simulink model "FinalShape"  (R2020a)
settings: Solver=ode4  StartTime=0.0  StopTime=100  FixedStep=.0001  MaxStep=1e-4  RelTol=1e-3
undefined symbols (not defined in the file or in its folder): kappa_lut_axis, lut_cooling_T, lut_heating_T, sigbuilder_block
settings Model: Creator=nnnmmm  LastModifiedBy=nnnmmm
settings DataIOCC: ExternalInput=sim_input_T

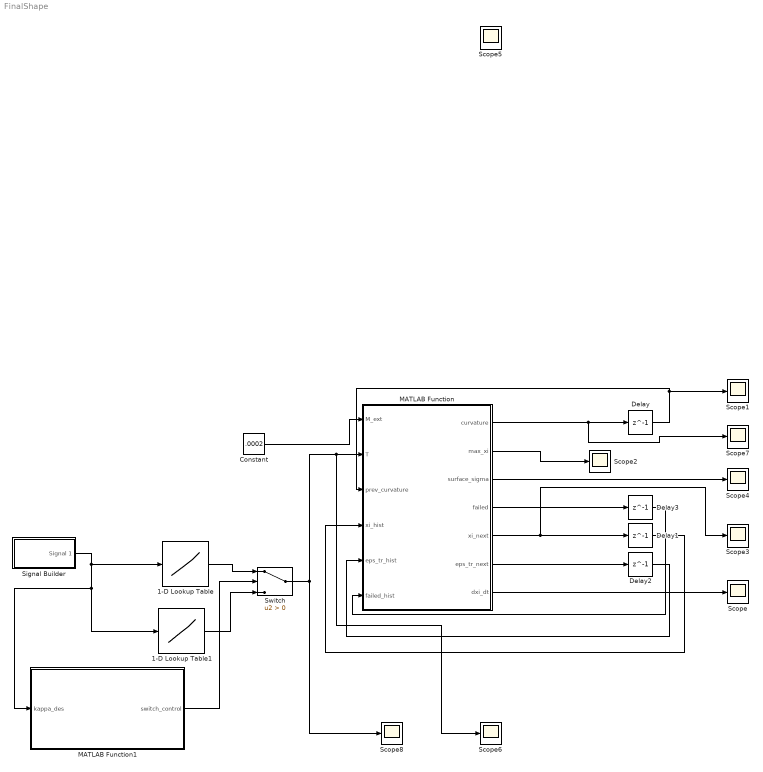
== system FinalShape ==
  1-D Lookup Table : Lookup_n-D  NumberOfTableDimensions=1  BreakpointsForDimension1=kappa_lut_axis  Table=lut_cooling_T  ExtrapMethod=Clip  InternalRulePriority=Speed  RndMeth=Simplest  InputSameDT=on
  1-D Lookup Table1 : Lookup_n-D  NumberOfTableDimensions=1  BreakpointsForDimension1=kappa_lut_axis  Table=lut_heating_T  ExtrapMethod=Clip  InternalRulePriority=Speed  RndMeth=Simplest  InputSameDT=on
  Constant : Constant  Value=.0002
  Delay : Delay  DelayLength=1
  Delay1 : Delay  DelayLength=1  InitialCondition=ones(1,11)
  Delay2 : Delay  DelayLength=1  InitialCondition=zeros(1,11)
  Delay3 : Delay  DelayLength=1
  MATLAB Function : MATLAB Function  TreatAsAtomicUnit=on
  MATLAB Function1 : MATLAB Function  TreatAsAtomicUnit=on
  Scope{,1..8} (9 alike) : Scope
  Signal Builder : Subsystem  Tag=STV Subsys  LoadFcn=sigbuilder_block('load');  StartFcn=sigbuilder_block('start');  StopFcn=sigbuilder_block('stop');  ClipboardFcn=sigbuilder_block('clipboard');  mask(Sigbuilder block){tuvar=[0:10]}
      mask help: Simulink:masks:SigbuilderBlock_MD
      mask init:
      | if ~strcmp(get_param(bdroot(gcbh),'SimulationStatus'),'stopped') tuvar = sigbuilder_block('maskInit'); end
      settings: CopyFcn=sigbuilder_block('copy');  DeleteFcn=sigbuilder_block('delete');  ModelCloseFcn=sigbuilder_block('modelClose');  PreSaveFcn=sigbuilder_block('preSave');  PauseFcn=sigbuilder_block('pause');  ContinueFcn=sigbuilder_block('continue');  NameChangeFcn=sigbuilder_block('namechange');  OpenFcn=sigbuilder_block('open',[5.4 36 1141.2 516.6 ]);  CloseFcn=sigbuilder_block('close');
      mask Display: plot(0, 0, 100, 100,[2, 2, 32, 32, 2], [68, 8, 8, 68, 68],[32, 2], [38, 38], [32, 19, 2],[53, 60, 44], [32, 17, 17, 2],[16, 16, 31, 31]);txt = getActiveGroup(gcbh);text(2, 100, txt,'verticalAlignment', 'top');
  Switch : Switch  Criteria=u2 > Threshold
  wires:
  Delay2/1 -> MATLAB Function/5(eps_tr_hist)
  MATLAB Function/6(eps_tr_next) -> Delay2/1
  MATLAB Function/1(curvature) -> Scope7/1, Delay/1
  MATLAB Function/4(failed) -> Delay3/1
  MATLAB Function/5(xi_next) -> Scope3/1, Delay1/1
  Delay/1 -> MATLAB Function/3(prev_curvature), Scope1/1
  Delay3/1 -> MATLAB Function/6(failed_hist)
  Delay1/1 -> MATLAB Function/4(xi_hist)
  Constant/1 -> MATLAB Function/1(M_ext)
  MATLAB Function/2(max_xi) -> Scope2/1
  MATLAB Function/7(dxi_dt) -> Scope/1
  MATLAB Function/3(surface_sigma) -> Scope4/1
  1-D Lookup Table1/1 -> Switch/3
  1-D Lookup Table/1 -> Switch/1
  Switch/1 -> Scope8/1, Scope6/1, MATLAB Function/2(T)
  MATLAB Function1/1(switch_control) -> Switch/2
  Signal Builder/1(Signal 1) -> 1-D Lookup Table/1, 1-D Lookup Table1/1, MATLAB Function1/1(kappa_des)

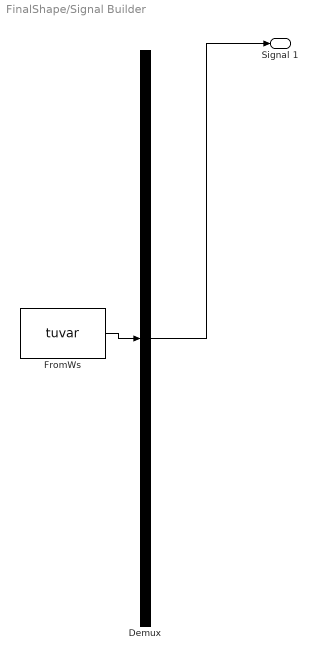
== system FinalShape/Signal Builder ==
  Demux : Demux  Tag=STV Demux  Outputs=1
      settings: DisplayOption=none
  FromWs : FromWorkspace  Tag=STV FromWs  VariableName=tuvar
      SigBuilderData=|
      | common.afterFinalStr = 'Extrapolate'
      | common.sampleTime = 0
      | dataSet.timeRange = [0 60]
      | dataSet.name = 'Group 1'
      | sbobj.Groups.Name = 'Group 1'
      | sbobj.Groups.Signals.Name = 'Signal 1'
      | sbobj.Groups.Signals.XData = [0 15 15 40 40 60]
      | sbobj.Groups.Signals.YData = [70 70 60 60 55 55]
      | sbobj.Groups.TimeRange = [0 60]
  Signal 1 : Outport  Tag=STV Outport
  wires:
  FromWs/1 -> Demux/1
  Demux/1 -> Signal 1/1

== matlab function FinalShape/MATLAB Function1 ==
  data: kappa_des input; switch_control output
function switch_control = direction_memory(kappa_des)
    % This persistent memory remembers the last direction permanently
    persistent last_state prev_kappa
    
    if isempty(last_state)
        last_state = -1;       % Start default: Heating table active
        prev_kappa = kappa_des; % Initialize tracking history
    end
    
    % Calculate the active change change
    delta = kappa_des - prev_kappa;
    
    if delta > 0.001
        last_state = 1;   % Target rose -> Lock onto Cooling table (u2 > 0)
    elseif delta < -0.001
        last_state = -1;  % Target dropped -> Lock onto Heating table (u2 < 0)
    end
    
    % Output stays locked at either -1 or 1 during all flat hold periods
    switch_control = last_state;
    prev_kappa = kappa_des;
end

== matlab function FinalShape/MATLAB Function ==
  data: M_ext input; T input; prev_curvature input; xi_hist input; eps_tr_hist input; curvature output; max_xi output; surface_sigma output; failed_hist input; failed output; xi_next output; eps_tr_next output; dxi_dt output
function [curvature, max_xi, surface_sigma, failed, xi_next, eps_tr_next, dxi_dt] = lagoudas_wire_pure_bending(M_ext , T, prev_curvature, xi_hist, eps_tr_hist, failed_hist)
%#codegen

% =========================================================================
% ─── SIMULINK CODER INCLUSIONS: IMMEDIATE VARIABLE INITIALIZATION ───
% =========================================================================
failed = failed_hist; % FIX: Inherit historical failure state immediately
curvature = prev_curvature;
max_xi = 0.0;
surface_sigma = 0.0;
dxi_dt = 0.0; 

% Strict [11 x 1] column vector properties for code generation alignment
xi_next = zeros(11, 1);
eps_tr_next = zeros(11, 1);

% Early exit if the wire has already failed historically
if failed_hist > 0.5
    failed = 1.0;
    return;
end

% =========================================================================
% 1. WIRE CROSS-SECTIONAL SLICE DISCRETIZATION (11 Symmetrical Layers)
% =========================================================================
R_wire = 0.25e-3;   
N_layers = 11;      
y_coords = linspace(-R_wire, R_wire, N_layers); 
y_coords = y_coords(:); 
dy = y_coords(2) - y_coords(1);
dt = 0.0001;        

xi_current = xi_hist(:);
eps_tr_current = eps_tr_hist(:);

% =========================================================================
% 2. EXPLICIT MATERIAL LITERAL CONSTANTS
% =========================================================================
E_A = 70e9;             
E_M = 30e9;             
H_max = 0.045;          
sigma_failure = 1000e6; 

Ms = 275; Mf = 256; As = 280; Af = 300; % Ms updated to 280 K
C_A = 8e6; C_M = 8e6;   
n1 = 2.0; n2 = 2.0; n3 = 2.0; n4 = 2.0; 

S_A = 1 / E_A; S_M = 1 / E_M; Delta_S = S_M - S_A; 

w_layer = 2 * sqrt(max(0, R_wire^2 - y_coords.^2));
dA = w_layer * dy;
S_curr_static = S_A + xi_current * Delta_S;

% =========================================================================
% 3. VECTORIZED EXPLICIT STATIC SOLVER LOOP FOR MECHANICAL EQUILIBRIUM
% =========================================================================
low_k = -150.0; 
high_k = 150.0; 
tol = 1e-6;
curvature = prev_curvature;
residual_mid = 0.0;

for iter = 1:60
    mid_k = (low_k + high_k) / 2;
    
    % Evaluate midpoint state residual
    eps_mid = -y_coords * mid_k;
    sigma_mid = (eps_mid - eps_tr_current) ./ S_curr_static;
    M_calc_mid = sum(-sigma_mid .* y_coords .* dA);
    residual_mid = M_calc_mid - M_ext;
    
    % Evaluate low-point state residual dynamically inside the loop
    % FIX: This forces the boundary checks to update with each step
    eps_low = -y_coords * low_k;
    sigma_low = (eps_low - eps_tr_current) ./ S_curr_static;
    M_calc_low = sum(-sigma_low .* y_coords .* dA);
    residual_low = M_calc_low - M_ext;
    
    if abs(residual_mid) < tol
        curvature = mid_k;
        break;
    end
    
    if (residual_low * residual_mid) < 0
        high_k = mid_k;
    else
        low_k = mid_k;
    end
end

if abs(residual_mid) >= tol
    curvature = (low_k + high_k) / 2;
end

% =========================================================================
% 4. LAYER PROGRESSION UPDATE WITH EXPLICIT RELAXATION FILTERING
% =========================================================================
sigma_max_track = 0.0;
xi_unfiltered = zeros(N_layers, 1);

for j = 1:N_layers
    epsilon = -y_coords(j) * curvature;
    S_curr = S_A + xi_current(j) * Delta_S;
    sigma_layer = (epsilon - eps_tr_current(j)) / S_curr;
    
    if abs(sigma_layer) > sigma_max_track
        sigma_max_track = abs(sigma_layer);
    end
    
    sgn_sig = sign(sigma_layer);
    if sgn_sig == 0; sgn_sig = 1; end
    
    Ms_s = Ms + abs(sigma_layer) / C_M;
    Mf_s = Mf + abs(sigma_layer) / C_M;
    As_s = As + abs(sigma_layer) / C_A;
    Af_s = Af + abs(sigma_layer) / C_A;
    
    xi_target = xi_current(j); 
    
    if abs(curvature) > 0.005
        if (T < Ms_s) && (T > Mf_s)
            linear_ratio = (T - Mf_s) / (Ms_s - Mf_s);
            trial_target = 1.0 - (linear_ratio^n1 / (linear_ratio^n1 + (1.0 - linear_ratio)^n2));
            if trial_target > xi_current(j); xi_target = trial_target; end
        elseif T <= Mf_s
            xi_target = 1.0;
        end
        
        if (T > As_s) && (T < Af_s)
            linear_ratio = (T - As_s) / (Af_s - As_s);
            trial_target = 1.0 - (linear_ratio^n3 / (linear_ratio^n3 + (1.0 - linear_ratio)^n4));
            if trial_target < xi_current(j); xi_target = trial_target; end
        elseif T >= Af_s
            xi_target = 0.0;
        end
    else
        if T > Af; xi_target = 0.0; elseif T < Mf; xi_target = 1.0; end
    end
    
    xi_unfiltered(j) = xi_target;
    
    % Balanced 5% relaxation factor
    xi_current(j) = xi_hist(j) + 0.05 * (xi_target - xi_hist(j));
    
    sigma_detwin = 70e6;
    if abs(sigma_layer) > 1e-3
        detwin_factor = min(1.0, abs(sigma_layer) / sigma_detwin);
        eps_tr_target = sgn_sig * H_max * xi_current(j) * detwin_factor;
    else
        eps_tr_target = 0.0;
    end
    
    eps_tr_current(j) = eps_tr_hist(j) + 0.05 * (eps_tr_target - eps_tr_hist(j));
end

if sigma_max_track > sigma_failure
    failed = 1.0;
end

% =========================================================================
% 5. ASSIGN FINAL OUTPUT PARAMETERS
% =========================================================================
max_xi = max(xi_current);
surface_sigma = sigma_max_track;

mean_xi_target = mean(xi_unfiltered);
mean_xi_hist = mean(xi_hist);
dxi_dt = (mean_xi_target - mean_xi_hist) / dt;

xi_next = xi_current(:);
eps_tr_next = eps_tr_current(:);

end
